simulink model "Torch_Bridge_Updated"  (R2020a)
settings: Solver=FixedStepAuto  StartTime=0.0  StopTime=10.0  FixedStep=1  RelTol=1e-3
undefined symbols (not defined in the file): sldvsubsys
libraries: sldvlib x1
settings Model: Creator=vivek vivian  LastModifiedBy=vivek vivian
settings ConfigComp: DVMode=PropertyProving  DVTestSuiteOptimization=Auto  DVDetectOutOfBounds=on

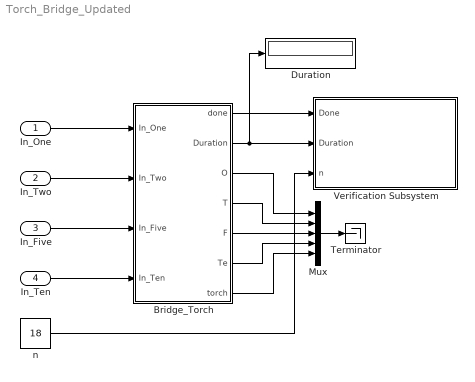
== system Torch_Bridge_Updated ==
  In_One : Inport
  In_Two : Inport  Port=2
  In_Five : Inport  Port=3
  In_Ten : Inport  Port=4
  Bridge_Torch : Stateflow chart  TreatAsAtomicUnit=on
  Duration : Display
  Mux : Mux  Inputs=5
  Terminator : Terminator
  Verification Subsystem : Subsystem  Tag=VerificationSubsystem  DisableCoverage=on  LoadFcn=sldvsubsys('check')  TreatAsAtomicUnit=on  SimViewingDevice=on  mask(VerificationSubsystem){}
      mask init:
      | sldvsubsys('maskInit');
      settings: CopyFcn=sldvsubsys('copy');  OpenFcn=open_system(gcb,'force');
      settings: PreSaveFcn=|
      | set_param(gcb,'SimViewingDevice','on');
      | sldvsubsys('check');
      mask Help: helpview(fullfile(docroot,'toolbox','sldv','sldv.map'),'verificationsubsystem')
      mask Display: image(imread('sldvicon_versubsys.png','BackGroundColor',[1 1 1]),'center');
  n : Constant  Value=18
  wires:
  In_Two/1 -> Bridge_Torch/2(In_Two)
  In_Five/1 -> Bridge_Torch/3(In_Five)
  In_Ten/1 -> Bridge_Torch/4(In_Ten)
  In_One/1 -> Bridge_Torch/1(In_One)
  Bridge_Torch/1(done) -> Verification Subsystem/1(Done)
  Bridge_Torch/2(Duration) -> Duration/1, Verification Subsystem/2(Duration)
  n/1 -> Verification Subsystem/3(n)
  Bridge_Torch/3(O) -> Mux/1
  Bridge_Torch/4(T) -> Mux/2
  Bridge_Torch/5(F) -> Mux/3
  Bridge_Torch/6(Te) -> Mux/4
  Mux/1 -> Terminator/1
  Bridge_Torch/7(torch) -> Mux/5

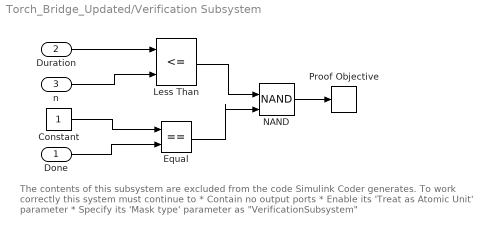
== system Torch_Bridge_Updated/Verification Subsystem ==
  note: The contents of this subsystem are excluded from the code Simulink Coder
      | generates.
      |
      | To work correctly this system must continue to
      | * Contain no output ports
      | * Enable its 'Treat as Atomic Unit' parameter
      | * Specify its 'Mask type' parameter as "VerificationSubsystem"
  Done : Inport
  Duration : Inport  Port=2
  n : Inport  Port=3
  Constant : Constant
  Equal : RelationalOperator  Operator===  OutDataTypeStr=boolean  RndMeth=Simplest
  Less Than : RelationalOperator  Operator=<=  OutDataTypeStr=boolean  RndMeth=Simplest
  NAND : Logic  Operator=NAND  IconShape=distinctive  AllPortsSameDT=off  OutDataTypeStr=boolean
  Proof Objective : sldvlib/Objectives and Constraints/Proof Objective  enabled=on  customAVTBlockType=Proof Objective  intervals=true  dispValues=on  outEnabled=off  enableStopSim=off
      settings: AttributesFormatString=%<intervals>  SourceProductBaseCode=SL
  wires:
  Duration/1 -> Less Than/1
  n/1 -> Less Than/2
  Done/1 -> Equal/2
  Constant/1 -> Equal/1
  Equal/1 -> NAND/2
  Less Than/1 -> NAND/1
  NAND/1 -> Proof Objective/1

== stateflow chart Torch_Bridge_Updated/Bridge_Torch ==
  settings: executeAtInitialization=1
  state Side_A
  state Destination
  (default) -> Side_A : {O=0;T=0;F=0;Te=0;done=0;torch=0;Tick=0;Duration=0;}
  Side_A -> (junction 129) : {criteria()}
  (junction 129) -> (junction 124) [order 2]
  (junction 129) -> (junction 124) [order 1] : [In_One && O==torch]{O=!O;Tick=1;}
  (junction 124) -> (junction 118) [order 1] : [In_Two && T==torch]{T=!T;Tick=2;}
  (junction 124) -> (junction 118) [order 2]
  (junction 118) -> (junction 121) [order 2]
  (junction 118) -> (junction 121) [order 1] : [In_Five && F==torch]{F=!F;Tick=5;}
  (junction 121) -> (junction 117) [order 2]
  (junction 121) -> (junction 117) [order 1] : [In_Ten && Te==torch]{Te=!Te;Tick=10;}
  (junction 117) -> (junction 130) : {Duration=Duration+Tick;}
  (junction 130) -> Side_A [order 2] : {torch=!torch;Tick=0;}
  (junction 130) -> Destination [order 1] : [O==1 && T==1 && F==1 && Te==1]{done=1}
  data: In_One input boolean; In_Two input boolean; In_Five input boolean; In_Ten input boolean; done output boolean; Tick local double; Duration output double; O output boolean; T output boolean; F output boolean; Te output boolean; torch output boolean
  function criteria:
    | function criteria()
    | sldv.assume(In_One+In_Two+In_Five+In_Ten <= 2);
    | sldv.assume(In_One+In_Two+In_Five+In_Ten > 0);
    | sldv.assume((In_One && O==torch) || (In_Two && T==torch) || (In_Five && F==torch)|| (In_Ten && Te==torch));
    | end
